simulink model "HANcoder_E407_TTA_Template_DS_V52"  (R2023a)
settings: Solver=FixedStepDiscrete  StartTime=0.0  StopTime=1  FixedStep=0.01  RelTol=1e-3
PreLoadFcn:
  | librarySetup
  | eval([bdroot,'_startup']) %Calling [modelName]_startup.m
values from neighbouring files (symbols this model uses):
  basic_cycle_duration_bc0 = TM_Reset_Board   + COMP_duration    (= 372)    [HANcoder_E407_TTA_Template_DS_V1_startup.m]    (also in HANcoder_E407_TTA_Template_DS_V2_startup.m; HANcoder_E407_TTA_Template_DS_V52_startup.m; HANcoder_E407_TTA_Template_DS_V5_startup.m; HANcoder_E407_TTA_Template_DS_V6_startup.m = 532)
  basic_cycle_duration_bc1 = basic_cycle_duration_bc0    (= 372)    [HANcoder_E407_TTA_Template_DS_V1_startup.m]    (also in HANcoder_E407_TTA_Template_DS_V2_startup.m; HANcoder_E407_TTA_Template_DS_V52_startup.m; HANcoder_E407_TTA_Template_DS_V5_startup.m; HANcoder_E407_TTA_Template_DS_V6_startup.m = 532)
  basic_cycle_duration_bc2 = basic_cycle_duration_bc0    (= 372)    [HANcoder_E407_TTA_Template_DS_V1_startup.m]    (also in HANcoder_E407_TTA_Template_DS_V2_startup.m; HANcoder_E407_TTA_Template_DS_V52_startup.m; HANcoder_E407_TTA_Template_DS_V5_startup.m; HANcoder_E407_TTA_Template_DS_V6_startup.m = 532)
  comm_delay_estimation1 = round(comm_delay_measured1*hardware_granularity/frequency_IRQ)    [HANcoder_E407_TTA_Template_DS_V1_startup.m]    (also in HANcoder_E407_TTA_Template_DS_V2_startup.m; HANcoder_E407_TTA_Template_DS_V52_startup.m; HANcoder_E407_TTA_Template_DS_V5_startup.m; HANcoder_E407_TTA_Template_DS_V6_startup.m)
  comm_delay_estimation2 = round(comm_delay_measured2*hardware_granularity/frequency_IRQ)    [HANcoder_E407_TTA_Template_DS_V1_startup.m]    (also in HANcoder_E407_TTA_Template_DS_V2_startup.m; HANcoder_E407_TTA_Template_DS_V52_startup.m; HANcoder_E407_TTA_Template_DS_V5_startup.m; HANcoder_E407_TTA_Template_DS_V6_startup.m)
  COMM_Period = 80    [HANcoder_E407_TTA_Template_DS_V1_startup.m]    (also in HANcoder_E407_TTA_Template_DS_V2_startup.m; HANcoder_E407_TTA_Template_DS_V52_startup.m; HANcoder_E407_TTA_Template_DS_V5_startup.m; HANcoder_E407_TTA_Template_DS_V6_startup.m = 120)
  COMM_Phase1 = Simulink.Parameter    [HANcoder_E407_TTA_Template_DS_V1_startup.m]    (also in HANcoder_E407_TTA_Template_DS_V2_startup.m; HANcoder_E407_TTA_Template_DS_V52_startup.m; HANcoder_E407_TTA_Template_DS_V5_startup.m; HANcoder_E407_TTA_Template_DS_V6_startup.m)
  COMM_Phase2 = Simulink.Parameter    [HANcoder_E407_TTA_Template_DS_V1_startup.m]    (also in HANcoder_E407_TTA_Template_DS_V2_startup.m; HANcoder_E407_TTA_Template_DS_V52_startup.m; HANcoder_E407_TTA_Template_DS_V5_startup.m; HANcoder_E407_TTA_Template_DS_V6_startup.m)
  COMM_Phase_init1 = Simulink.Parameter    [HANcoder_E407_TTA_Template_DS_V1_startup.m]    (also in HANcoder_E407_TTA_Template_DS_V2_startup.m; HANcoder_E407_TTA_Template_DS_V52_startup.m; HANcoder_E407_TTA_Template_DS_V5_startup.m; HANcoder_E407_TTA_Template_DS_V6_startup.m)
  COMM_Phase_init2 = Simulink.Parameter    [HANcoder_E407_TTA_Template_DS_V1_startup.m]    (also in HANcoder_E407_TTA_Template_DS_V2_startup.m; HANcoder_E407_TTA_Template_DS_V52_startup.m; HANcoder_E407_TTA_Template_DS_V5_startup.m; HANcoder_E407_TTA_Template_DS_V6_startup.m)
  COMP_duration = 4    [HANcoder_E407_TTA_Template_DS_V1_startup.m]    (also in HANcoder_E407_TTA_Template_DS_V2_startup.m; HANcoder_E407_TTA_Template_DS_V52_startup.m; HANcoder_E407_TTA_Template_DS_V5_startup.m; HANcoder_E407_TTA_Template_DS_V6_startup.m)
  frequency_IRQ = 100    [HANcoder_E407_TTA_Template_DS_V1_startup.m]    (also in HANcoder_E407_TTA_Template_DS_V2_startup.m; HANcoder_E407_TTA_Template_DS_V52_startup.m; HANcoder_E407_TTA_Template_DS_V5_startup.m; HANcoder_E407_TTA_Template_DS_V6_startup.m)
  idle_time_init = basic_cycle_duration_bc0 + basic_cycle_duration_bc1    (= 744)    [HANcoder_E407_TTA_Template_DS_V1_startup.m]    (also in HANcoder_E407_TTA_Template_DS_V2_startup.m; HANcoder_E407_TTA_Template_DS_V52_startup.m = 1116; HANcoder_E407_TTA_Template_DS_V5_startup.m = 1116; HANcoder_E407_TTA_Template_DS_V6_startup.m = 1596)
  L0b = 0.5    [HANcoder_E407_TTA_Template_DS_V52_startup.m]    (also in HANcoder_E407_TTA_Template_DS_V5_startup.m; HANcoder_E407_TTA_Template_DS_V6_startup.m)
  L0f = 5    [HANcoder_E407_TTA_Template_DS_V52_startup.m]    (also in HANcoder_E407_TTA_Template_DS_V5_startup.m; HANcoder_E407_TTA_Template_DS_V6_startup.m)
  L1f = 6    [HANcoder_E407_TTA_Template_DS_V52_startup.m]    (also in HANcoder_E407_TTA_Template_DS_V5_startup.m; HANcoder_E407_TTA_Template_DS_V6_startup.m)
  LA_Clock_Gr = 1    [HANcoder_E407_TTA_Template_DS_V1_startup.m]    (also in HANcoder_E407_TTA_Template_DS_V2_startup.m; HANcoder_E407_TTA_Template_DS_V52_startup.m; HANcoder_E407_TTA_Template_DS_V5_startup.m; HANcoder_E407_TTA_Template_DS_V6_startup.m)
  LA_COMM_dly = 1    [HANcoder_E407_TTA_Template_DS_V1_startup.m]    (also in HANcoder_E407_TTA_Template_DS_V2_startup.m; HANcoder_E407_TTA_Template_DS_V52_startup.m; HANcoder_E407_TTA_Template_DS_V5_startup.m; HANcoder_E407_TTA_Template_DS_V6_startup.m)
  LA_COMM_Err = 1    [HANcoder_E407_TTA_Template_DS_V1_startup.m]    (also in HANcoder_E407_TTA_Template_DS_V2_startup.m; HANcoder_E407_TTA_Template_DS_V52_startup.m; HANcoder_E407_TTA_Template_DS_V5_startup.m; HANcoder_E407_TTA_Template_DS_V6_startup.m)
  LA_E_Desync = 1    [HANcoder_E407_TTA_Template_DS_V1_startup.m]    (also in HANcoder_E407_TTA_Template_DS_V2_startup.m; HANcoder_E407_TTA_Template_DS_V52_startup.m; HANcoder_E407_TTA_Template_DS_V5_startup.m; HANcoder_E407_TTA_Template_DS_V6_startup.m)
  LA_MEX_Flag = 1    [HANcoder_E407_TTA_Template_DS_V1_startup.m]    (also in HANcoder_E407_TTA_Template_DS_V2_startup.m; HANcoder_E407_TTA_Template_DS_V52_startup.m; HANcoder_E407_TTA_Template_DS_V5_startup.m; HANcoder_E407_TTA_Template_DS_V6_startup.m)
  LA_Task_Act = 1    [HANcoder_E407_TTA_Template_DS_V1_startup.m]    (also in HANcoder_E407_TTA_Template_DS_V2_startup.m; HANcoder_E407_TTA_Template_DS_V52_startup.m; HANcoder_E407_TTA_Template_DS_V5_startup.m; HANcoder_E407_TTA_Template_DS_V6_startup.m)
  Master_Role = 1    [HANcoder_E407_TTA_Template_DS_V1_startup.m]    (also in HANcoder_E407_TTA_Template_DS_V2_startup.m; HANcoder_E407_TTA_Template_DS_V52_startup.m; HANcoder_E407_TTA_Template_DS_V5_startup.m; HANcoder_E407_TTA_Template_DS_V6_startup.m)
  matrix_rows = 3    [HANcoder_E407_TTA_Template_DS_V1_startup.m]    (also in HANcoder_E407_TTA_Template_DS_V2_startup.m; HANcoder_E407_TTA_Template_DS_V52_startup.m; HANcoder_E407_TTA_Template_DS_V5_startup.m; HANcoder_E407_TTA_Template_DS_V6_startup.m)
  max_desync = 15    [HANcoder_E407_TTA_Template_DS_V1_startup.m]    (also in HANcoder_E407_TTA_Template_DS_V2_startup.m; HANcoder_E407_TTA_Template_DS_V52_startup.m; HANcoder_E407_TTA_Template_DS_V5_startup.m; HANcoder_E407_TTA_Template_DS_V6_startup.m)
  max_num_msgs_CAN1 = 2^Tx_bit_number-1    (= 7)    [HANcoder_E407_TTA_Template_DS_V1_startup.m]    (also in HANcoder_E407_TTA_Template_DS_V2_startup.m; HANcoder_E407_TTA_Template_DS_V52_startup.m; HANcoder_E407_TTA_Template_DS_V5_startup.m; HANcoder_E407_TTA_Template_DS_V6_startup.m)
  max_num_msgs_CAN2 = max_num_msgs_CAN1    (= 7)    [HANcoder_E407_TTA_Template_DS_V1_startup.m]    (also in HANcoder_E407_TTA_Template_DS_V2_startup.m; HANcoder_E407_TTA_Template_DS_V52_startup.m; HANcoder_E407_TTA_Template_DS_V5_startup.m; HANcoder_E407_TTA_Template_DS_V6_startup.m)
  min_desync = (-1)*max_desync    (= -15)    [HANcoder_E407_TTA_Template_DS_V1_startup.m]    (also in HANcoder_E407_TTA_Template_DS_V2_startup.m; HANcoder_E407_TTA_Template_DS_V52_startup.m; HANcoder_E407_TTA_Template_DS_V5_startup.m; HANcoder_E407_TTA_Template_DS_V6_startup.m)
  PID_derivative = Simulink.Parameter    [HANcoder_E407_TTA_Template_DS_V52_startup.m]    (also in HANcoder_E407_TTA_Template_DS_V6_startup.m)
  PID_gain = Simulink.Parameter    [HANcoder_E407_TTA_Template_DS_V52_startup.m]    (also in HANcoder_E407_TTA_Template_DS_V6_startup.m)
  PID_integrator = Simulink.Parameter    [HANcoder_E407_TTA_Template_DS_V52_startup.m]    (also in HANcoder_E407_TTA_Template_DS_V6_startup.m)
  PotValue1_ID = 22    [HANcoder_E407_TTA_Template_DS_V1_startup.m]    (also in HANcoder_E407_TTA_Template_DS_V2_startup.m; HANcoder_E407_TTA_Template_DS_V52_startup.m; HANcoder_E407_TTA_Template_DS_V5_startup.m; HANcoder_E407_TTA_Template_DS_V6_startup.m)
  PotValue2_ID = 23    [HANcoder_E407_TTA_Template_DS_V1_startup.m]    (also in HANcoder_E407_TTA_Template_DS_V2_startup.m; HANcoder_E407_TTA_Template_DS_V52_startup.m; HANcoder_E407_TTA_Template_DS_V5_startup.m; HANcoder_E407_TTA_Template_DS_V6_startup.m)
  PotValue3_ID = 24    [HANcoder_E407_TTA_Template_DS_V1_startup.m]    (also in HANcoder_E407_TTA_Template_DS_V2_startup.m; HANcoder_E407_TTA_Template_DS_V52_startup.m; HANcoder_E407_TTA_Template_DS_V5_startup.m; HANcoder_E407_TTA_Template_DS_V6_startup.m)
  script_run = Simulink.Parameter    [HANcoder_E407_TTA_Template_DS_V1_startup.m]    (also in HANcoder_E407_TTA_Template_DS_V2_startup.m; HANcoder_E407_TTA_Template_DS_V52_startup.m; HANcoder_E407_TTA_Template_DS_V5_startup.m; HANcoder_E407_TTA_Template_DS_V6_startup.m)
  Slave_Role = 2    [HANcoder_E407_TTA_Template_DS_V1_startup.m]    (also in HANcoder_E407_TTA_Template_DS_V2_startup.m; HANcoder_E407_TTA_Template_DS_V52_startup.m; HANcoder_E407_TTA_Template_DS_V5_startup.m; HANcoder_E407_TTA_Template_DS_V6_startup.m)
  Sync_ID = 1    [HANcoder_E407_TTA_Template_DS_V1_startup.m]    (also in HANcoder_E407_TTA_Template_DS_V2_startup.m; HANcoder_E407_TTA_Template_DS_V52_startup.m; HANcoder_E407_TTA_Template_DS_V5_startup.m; HANcoder_E407_TTA_Template_DS_V6_startup.m)
  TM_Check_PotValue1 = TM_COMM_PotValue1 + COMM_duration    (= 174)    [HANcoder_E407_TTA_Template_DS_V1_startup.m]    (also in HANcoder_E407_TTA_Template_DS_V2_startup.m; HANcoder_E407_TTA_Template_DS_V52_startup.m; HANcoder_E407_TTA_Template_DS_V5_startup.m; HANcoder_E407_TTA_Template_DS_V6_startup.m = 254)
  TM_Check_PotValue2 = TM_COMM_PotValue2 + COMM_duration    (= 258)    [HANcoder_E407_TTA_Template_DS_V1_startup.m]    (also in HANcoder_E407_TTA_Template_DS_V2_startup.m; HANcoder_E407_TTA_Template_DS_V52_startup.m; HANcoder_E407_TTA_Template_DS_V5_startup.m; HANcoder_E407_TTA_Template_DS_V6_startup.m = 378)
  TM_Check_PotValue3 = TM_COMM_PotValue3 + COMM_duration    (= 342)    [HANcoder_E407_TTA_Template_DS_V1_startup.m]    (also in HANcoder_E407_TTA_Template_DS_V2_startup.m; HANcoder_E407_TTA_Template_DS_V52_startup.m; HANcoder_E407_TTA_Template_DS_V5_startup.m; HANcoder_E407_TTA_Template_DS_V6_startup.m = 502)
  TM_Check_Sync = TM_COMM_Sync   + COMM_duration    (= 80)    [HANcoder_E407_TTA_Template_DS_V1_startup.m]    (also in HANcoder_E407_TTA_Template_DS_V2_startup.m; HANcoder_E407_TTA_Template_DS_V52_startup.m; HANcoder_E407_TTA_Template_DS_V5_startup.m; HANcoder_E407_TTA_Template_DS_V6_startup.m = 120)
  TM_Check_TOuts = TM_Count_Vote3 + COMP_duration    (= 356)    [HANcoder_E407_TTA_Template_DS_V1_startup.m]    (also in HANcoder_E407_TTA_Template_DS_V2_startup.m; HANcoder_E407_TTA_Template_DS_V52_startup.m; HANcoder_E407_TTA_Template_DS_V5_startup.m; HANcoder_E407_TTA_Template_DS_V6_startup.m = 516)
  TM_Check_Trailer1Articulation = TM_COMM_Trailer1Articulation + COMM_duration    (= 170)    [HANcoder_E407_TTA_Template_DS_V1_startup.m]    (also in HANcoder_E407_TTA_Template_DS_V2_startup.m; HANcoder_E407_TTA_Template_DS_V52_startup.m; HANcoder_E407_TTA_Template_DS_V5_startup.m; HANcoder_E407_TTA_Template_DS_V6_startup.m = 250)
  TM_Check_Trailer2Articulation = TM_COMM_Trailer2Articulation + COMM_duration    (= 254)    [HANcoder_E407_TTA_Template_DS_V1_startup.m]    (also in HANcoder_E407_TTA_Template_DS_V2_startup.m; HANcoder_E407_TTA_Template_DS_V52_startup.m; HANcoder_E407_TTA_Template_DS_V5_startup.m; HANcoder_E407_TTA_Template_DS_V6_startup.m = 374)
  TM_Check_Vote1 = TM_COMM_Vote1  + COMM_duration    (= 172)    [HANcoder_E407_TTA_Template_DS_V1_startup.m]    (also in HANcoder_E407_TTA_Template_DS_V2_startup.m; HANcoder_E407_TTA_Template_DS_V52_startup.m; HANcoder_E407_TTA_Template_DS_V5_startup.m; HANcoder_E407_TTA_Template_DS_V6_startup.m = 252)
  TM_Check_Vote2 = TM_COMM_Vote2  + COMM_duration    (= 260)    [HANcoder_E407_TTA_Template_DS_V1_startup.m]    (also in HANcoder_E407_TTA_Template_DS_V2_startup.m; HANcoder_E407_TTA_Template_DS_V52_startup.m; HANcoder_E407_TTA_Template_DS_V5_startup.m; HANcoder_E407_TTA_Template_DS_V6_startup.m = 380)
  TM_Check_Vote3 = TM_COMM_Vote3  + COMM_duration    (= 348)    [HANcoder_E407_TTA_Template_DS_V1_startup.m]    (also in HANcoder_E407_TTA_Template_DS_V2_startup.m; HANcoder_E407_TTA_Template_DS_V52_startup.m; HANcoder_E407_TTA_Template_DS_V5_startup.m; HANcoder_E407_TTA_Template_DS_V6_startup.m = 508)
  TM_COMM_PotValue1 = TM_ReadPot + COMP_duration    (= 94)    [HANcoder_E407_TTA_Template_DS_V1_startup.m]    (also in HANcoder_E407_TTA_Template_DS_V2_startup.m; HANcoder_E407_TTA_Template_DS_V52_startup.m; HANcoder_E407_TTA_Template_DS_V5_startup.m; HANcoder_E407_TTA_Template_DS_V6_startup.m = 134)
  TM_COMM_PotValue2 = TM_Check_PotValue1 + COMP_duration    (= 178)    [HANcoder_E407_TTA_Template_DS_V1_startup.m]    (also in HANcoder_E407_TTA_Template_DS_V2_startup.m; HANcoder_E407_TTA_Template_DS_V52_startup.m; HANcoder_E407_TTA_Template_DS_V5_startup.m; HANcoder_E407_TTA_Template_DS_V6_startup.m = 258)
  TM_COMM_PotValue3 = TM_Check_PotValue2 + COMP_duration    (= 262)    [HANcoder_E407_TTA_Template_DS_V1_startup.m]    (also in HANcoder_E407_TTA_Template_DS_V2_startup.m; HANcoder_E407_TTA_Template_DS_V52_startup.m; HANcoder_E407_TTA_Template_DS_V5_startup.m; HANcoder_E407_TTA_Template_DS_V6_startup.m = 382)
  TM_COMM_Sync = basic_cycle_start    (= 0)    [HANcoder_E407_TTA_Template_DS_V1_startup.m]    (also in HANcoder_E407_TTA_Template_DS_V2_startup.m; HANcoder_E407_TTA_Template_DS_V52_startup.m; HANcoder_E407_TTA_Template_DS_V5_startup.m; HANcoder_E407_TTA_Template_DS_V6_startup.m)
  TM_COMM_Trailer1Articulation = TM_Update_LT_2 + COMP_duration    (= 90)    [HANcoder_E407_TTA_Template_DS_V1_startup.m]    (also in HANcoder_E407_TTA_Template_DS_V2_startup.m; HANcoder_E407_TTA_Template_DS_V52_startup.m; HANcoder_E407_TTA_Template_DS_V5_startup.m; HANcoder_E407_TTA_Template_DS_V6_startup.m = 130)
  TM_COMM_Trailer2Articulation = TM_Check_Trailer1Articulation + COMP_duration    (= 174)    [HANcoder_E407_TTA_Template_DS_V1_startup.m]    (also in HANcoder_E407_TTA_Template_DS_V2_startup.m; HANcoder_E407_TTA_Template_DS_V52_startup.m; HANcoder_E407_TTA_Template_DS_V5_startup.m; HANcoder_E407_TTA_Template_DS_V6_startup.m = 254)
  TM_COMM_Vote1 = TM_Vote_Dec    + COMP_duration    (= 92)    [HANcoder_E407_TTA_Template_DS_V1_startup.m]    (also in HANcoder_E407_TTA_Template_DS_V2_startup.m; HANcoder_E407_TTA_Template_DS_V52_startup.m; HANcoder_E407_TTA_Template_DS_V5_startup.m; HANcoder_E407_TTA_Template_DS_V6_startup.m = 132)
  TM_COMM_Vote2 = TM_Count_Vote1 + COMP_duration    (= 180)    [HANcoder_E407_TTA_Template_DS_V1_startup.m]    (also in HANcoder_E407_TTA_Template_DS_V2_startup.m; HANcoder_E407_TTA_Template_DS_V52_startup.m; HANcoder_E407_TTA_Template_DS_V5_startup.m; HANcoder_E407_TTA_Template_DS_V6_startup.m = 260)
  TM_COMM_Vote3 = TM_Count_Vote2 + COMP_duration    (= 268)    [HANcoder_E407_TTA_Template_DS_V1_startup.m]    (also in HANcoder_E407_TTA_Template_DS_V2_startup.m; HANcoder_E407_TTA_Template_DS_V52_startup.m; HANcoder_E407_TTA_Template_DS_V5_startup.m; HANcoder_E407_TTA_Template_DS_V6_startup.m = 388)
  TM_Count_Vote1 = TM_Check_Vote1 + COMP_duration    (= 176)    [HANcoder_E407_TTA_Template_DS_V1_startup.m]    (also in HANcoder_E407_TTA_Template_DS_V2_startup.m; HANcoder_E407_TTA_Template_DS_V52_startup.m; HANcoder_E407_TTA_Template_DS_V5_startup.m; HANcoder_E407_TTA_Template_DS_V6_startup.m = 256)
  TM_Count_Vote2 = TM_Check_Vote2 + COMP_duration    (= 264)    [HANcoder_E407_TTA_Template_DS_V1_startup.m]    (also in HANcoder_E407_TTA_Template_DS_V2_startup.m; HANcoder_E407_TTA_Template_DS_V52_startup.m; HANcoder_E407_TTA_Template_DS_V5_startup.m; HANcoder_E407_TTA_Template_DS_V6_startup.m = 384)
  TM_Count_Vote3 = TM_Check_Vote3 + COMP_duration    (= 352)    [HANcoder_E407_TTA_Template_DS_V1_startup.m]    (also in HANcoder_E407_TTA_Template_DS_V2_startup.m; HANcoder_E407_TTA_Template_DS_V52_startup.m; HANcoder_E407_TTA_Template_DS_V5_startup.m; HANcoder_E407_TTA_Template_DS_V6_startup.m = 512)
  TM_Data_bc0 = TM_COMM_Sync    (= 0)    [HANcoder_E407_TTA_Template_DS_V1_startup.m]    (also in HANcoder_E407_TTA_Template_DS_V2_startup.m; HANcoder_E407_TTA_Template_DS_V52_startup.m; HANcoder_E407_TTA_Template_DS_V5_startup.m; HANcoder_E407_TTA_Template_DS_V6_startup.m)
  TM_Data_bc1 = TM_Data_bc0(1:4)    [HANcoder_E407_TTA_Template_DS_V1_startup.m]    (also in HANcoder_E407_TTA_Template_DS_V2_startup.m; HANcoder_E407_TTA_Template_DS_V52_startup.m; HANcoder_E407_TTA_Template_DS_V5_startup.m; HANcoder_E407_TTA_Template_DS_V6_startup.m)
  TM_Data_bc2 = TM_Data_bc0(1:4)    [HANcoder_E407_TTA_Template_DS_V1_startup.m]    (also in HANcoder_E407_TTA_Template_DS_V2_startup.m; HANcoder_E407_TTA_Template_DS_V52_startup.m; HANcoder_E407_TTA_Template_DS_V5_startup.m; HANcoder_E407_TTA_Template_DS_V6_startup.m)
  TM_InverseKinematics = TM_Check_Trailer2Articulation + COMP_duration    (= 258)    [HANcoder_E407_TTA_Template_DS_V1_startup.m]    (also in HANcoder_E407_TTA_Template_DS_V2_startup.m; HANcoder_E407_TTA_Template_DS_V52_startup.m; HANcoder_E407_TTA_Template_DS_V5_startup.m; HANcoder_E407_TTA_Template_DS_V6_startup.m = 378)
  TM_New_Master = TM_Check_TOuts + COMP_duration    (= 360)    [HANcoder_E407_TTA_Template_DS_V1_startup.m]    (also in HANcoder_E407_TTA_Template_DS_V2_startup.m; HANcoder_E407_TTA_Template_DS_V52_startup.m; HANcoder_E407_TTA_Template_DS_V5_startup.m; HANcoder_E407_TTA_Template_DS_V6_startup.m = 520)
  TM_PotVote = TM_COMM_PotValue3 + COMP_duration    (= 266)    [HANcoder_E407_TTA_Template_DS_V1_startup.m]    (also in HANcoder_E407_TTA_Template_DS_V2_startup.m; HANcoder_E407_TTA_Template_DS_V52_startup.m; HANcoder_E407_TTA_Template_DS_V5_startup.m; HANcoder_E407_TTA_Template_DS_V6_startup.m = 386)
  TM_ReadPot = TM_Update_LT_2 + COMP_duration    (= 90)    [HANcoder_E407_TTA_Template_DS_V1_startup.m]    (also in HANcoder_E407_TTA_Template_DS_V2_startup.m; HANcoder_E407_TTA_Template_DS_V52_startup.m; HANcoder_E407_TTA_Template_DS_V5_startup.m; HANcoder_E407_TTA_Template_DS_V6_startup.m = 130)
  TM_Reset_Board = TM_Reset_Var   + COMP_duration    (= 368)    [HANcoder_E407_TTA_Template_DS_V1_startup.m]    (also in HANcoder_E407_TTA_Template_DS_V2_startup.m; HANcoder_E407_TTA_Template_DS_V52_startup.m; HANcoder_E407_TTA_Template_DS_V5_startup.m; HANcoder_E407_TTA_Template_DS_V6_startup.m = 528)
  TM_Reset_Var = TM_New_Master  + COMP_duration    (= 364)    [HANcoder_E407_TTA_Template_DS_V1_startup.m]    (also in HANcoder_E407_TTA_Template_DS_V2_startup.m; HANcoder_E407_TTA_Template_DS_V52_startup.m; HANcoder_E407_TTA_Template_DS_V5_startup.m; HANcoder_E407_TTA_Template_DS_V6_startup.m = 524)
  TM_Reset_Var_bc1 = TM_Data_bc1(end) + COMP_duration    [HANcoder_E407_TTA_Template_DS_V1_startup.m]    (also in HANcoder_E407_TTA_Template_DS_V2_startup.m; HANcoder_E407_TTA_Template_DS_V52_startup.m; HANcoder_E407_TTA_Template_DS_V5_startup.m; HANcoder_E407_TTA_Template_DS_V6_startup.m)
  TM_Reset_Var_bc1_2 = TM_Reset_Var_bc1 +2    [HANcoder_E407_TTA_Template_DS_V1_startup.m]    (also in HANcoder_E407_TTA_Template_DS_V2_startup.m; HANcoder_E407_TTA_Template_DS_V52_startup.m; HANcoder_E407_TTA_Template_DS_V5_startup.m; HANcoder_E407_TTA_Template_DS_V6_startup.m)
  TM_Reset_Var_bc2 = TM_Data_bc2(end) + COMP_duration    [HANcoder_E407_TTA_Template_DS_V1_startup.m]    (also in HANcoder_E407_TTA_Template_DS_V2_startup.m; HANcoder_E407_TTA_Template_DS_V52_startup.m; HANcoder_E407_TTA_Template_DS_V5_startup.m; HANcoder_E407_TTA_Template_DS_V6_startup.m)
  TM_Reset_Var_bc2_2 = TM_Reset_Var_bc2 +2    [HANcoder_E407_TTA_Template_DS_V1_startup.m]    (also in HANcoder_E407_TTA_Template_DS_V2_startup.m; HANcoder_E407_TTA_Template_DS_V52_startup.m; HANcoder_E407_TTA_Template_DS_V5_startup.m; HANcoder_E407_TTA_Template_DS_V6_startup.m)
  TM_SteerControl = TM_InverseKinematics + COMP_duration    (= 262)    [HANcoder_E407_TTA_Template_DS_V1_startup.m]    (also in HANcoder_E407_TTA_Template_DS_V2_startup.m; HANcoder_E407_TTA_Template_DS_V52_startup.m = 259; HANcoder_E407_TTA_Template_DS_V5_startup.m = 259)
  TM_Type_bc0 = COMM    (= 0)    [HANcoder_E407_TTA_Template_DS_V1_startup.m]    (also in HANcoder_E407_TTA_Template_DS_V2_startup.m; HANcoder_E407_TTA_Template_DS_V52_startup.m; HANcoder_E407_TTA_Template_DS_V5_startup.m; HANcoder_E407_TTA_Template_DS_V6_startup.m)
  TM_Type_bc1 = TM_Type_bc0(1:4)    [HANcoder_E407_TTA_Template_DS_V1_startup.m]    (also in HANcoder_E407_TTA_Template_DS_V2_startup.m; HANcoder_E407_TTA_Template_DS_V52_startup.m; HANcoder_E407_TTA_Template_DS_V5_startup.m; HANcoder_E407_TTA_Template_DS_V6_startup.m)
  TM_Type_bc2 = TM_Type_bc0(1:4)    [HANcoder_E407_TTA_Template_DS_V1_startup.m]    (also in HANcoder_E407_TTA_Template_DS_V2_startup.m; HANcoder_E407_TTA_Template_DS_V52_startup.m; HANcoder_E407_TTA_Template_DS_V5_startup.m; HANcoder_E407_TTA_Template_DS_V6_startup.m)
  TM_Update_LT = TM_Check_Sync  + COMP_duration    (= 84)    [HANcoder_E407_TTA_Template_DS_V1_startup.m]    (also in HANcoder_E407_TTA_Template_DS_V2_startup.m; HANcoder_E407_TTA_Template_DS_V52_startup.m; HANcoder_E407_TTA_Template_DS_V5_startup.m; HANcoder_E407_TTA_Template_DS_V6_startup.m = 124)
  TM_Update_LT_2 = TM_Update_LT   + 2    (= 86)    [HANcoder_E407_TTA_Template_DS_V1_startup.m]    (also in HANcoder_E407_TTA_Template_DS_V2_startup.m; HANcoder_E407_TTA_Template_DS_V52_startup.m; HANcoder_E407_TTA_Template_DS_V5_startup.m; HANcoder_E407_TTA_Template_DS_V6_startup.m = 126)
  TM_Vote_Dec = TM_Update_LT   + COMP_duration    (= 88)    [HANcoder_E407_TTA_Template_DS_V1_startup.m]    (also in HANcoder_E407_TTA_Template_DS_V2_startup.m; HANcoder_E407_TTA_Template_DS_V52_startup.m; HANcoder_E407_TTA_Template_DS_V5_startup.m; HANcoder_E407_TTA_Template_DS_V6_startup.m = 128)
  Tractor_Board1 = 11    [HANcoder_E407_TTA_Template_DS_V1_startup.m]    (also in HANcoder_E407_TTA_Template_DS_V2_startup.m = 1; HANcoder_E407_TTA_Template_DS_V52_startup.m = 1; HANcoder_E407_TTA_Template_DS_V5_startup.m = 1; HANcoder_E407_TTA_Template_DS_V6_startup.m = 1)
  Tractor_Board2 = 12    [HANcoder_E407_TTA_Template_DS_V1_startup.m]    (also in HANcoder_E407_TTA_Template_DS_V2_startup.m = 2; HANcoder_E407_TTA_Template_DS_V52_startup.m = 2; HANcoder_E407_TTA_Template_DS_V5_startup.m = 2; HANcoder_E407_TTA_Template_DS_V6_startup.m = 2)
  Tractor_Board3 = 13    [HANcoder_E407_TTA_Template_DS_V1_startup.m]    (also in HANcoder_E407_TTA_Template_DS_V2_startup.m = 3; HANcoder_E407_TTA_Template_DS_V52_startup.m = 3; HANcoder_E407_TTA_Template_DS_V5_startup.m = 3; HANcoder_E407_TTA_Template_DS_V6_startup.m = 3)
  Trailer1_Articulation_ID = 31    [HANcoder_E407_TTA_Template_DS_V1_startup.m]    (also in HANcoder_E407_TTA_Template_DS_V2_startup.m; HANcoder_E407_TTA_Template_DS_V52_startup.m; HANcoder_E407_TTA_Template_DS_V5_startup.m; HANcoder_E407_TTA_Template_DS_V6_startup.m)
  Trailer1_Board1 = 2    [HANcoder_E407_TTA_Template_DS_V1_startup.m]    (also in HANcoder_E407_TTA_Template_DS_V2_startup.m = 4; HANcoder_E407_TTA_Template_DS_V52_startup.m = 4; HANcoder_E407_TTA_Template_DS_V5_startup.m = 4; HANcoder_E407_TTA_Template_DS_V6_startup.m = 4)
  Trailer1_Board2 = 3    [HANcoder_E407_TTA_Template_DS_V1_startup.m]    (also in HANcoder_E407_TTA_Template_DS_V2_startup.m = 5; HANcoder_E407_TTA_Template_DS_V52_startup.m = 5; HANcoder_E407_TTA_Template_DS_V5_startup.m = 5; HANcoder_E407_TTA_Template_DS_V6_startup.m = 5)
  Trailer1_Board3 = 4    [HANcoder_E407_TTA_Template_DS_V1_startup.m]    (also in HANcoder_E407_TTA_Template_DS_V2_startup.m = 6; HANcoder_E407_TTA_Template_DS_V52_startup.m = 6; HANcoder_E407_TTA_Template_DS_V5_startup.m = 6; HANcoder_E407_TTA_Template_DS_V6_startup.m = 6)
  Trailer2_Articulation_ID = 32    [HANcoder_E407_TTA_Template_DS_V1_startup.m]    (also in HANcoder_E407_TTA_Template_DS_V2_startup.m; HANcoder_E407_TTA_Template_DS_V52_startup.m; HANcoder_E407_TTA_Template_DS_V5_startup.m; HANcoder_E407_TTA_Template_DS_V6_startup.m)
  Trailer2_Board1 = 5    [HANcoder_E407_TTA_Template_DS_V1_startup.m]    (also in HANcoder_E407_TTA_Template_DS_V2_startup.m = 7; HANcoder_E407_TTA_Template_DS_V52_startup.m = 7; HANcoder_E407_TTA_Template_DS_V5_startup.m = 7; HANcoder_E407_TTA_Template_DS_V6_startup.m = 7)
  Trailer2_Board2 = 6    [HANcoder_E407_TTA_Template_DS_V1_startup.m]    (also in HANcoder_E407_TTA_Template_DS_V2_startup.m = 8; HANcoder_E407_TTA_Template_DS_V52_startup.m = 8; HANcoder_E407_TTA_Template_DS_V5_startup.m = 8; HANcoder_E407_TTA_Template_DS_V6_startup.m = 8)
  Trailer2_Board3 = 7    [HANcoder_E407_TTA_Template_DS_V1_startup.m]    (also in HANcoder_E407_TTA_Template_DS_V2_startup.m = 9; HANcoder_E407_TTA_Template_DS_V52_startup.m = 9; HANcoder_E407_TTA_Template_DS_V5_startup.m = 9; HANcoder_E407_TTA_Template_DS_V6_startup.m = 9)
  V1 = -0.000000001    (= -1e-09)    [HANcoder_E407_TTA_Template_DS_V52_startup.m]    (also in HANcoder_E407_TTA_Template_DS_V5_startup.m; HANcoder_E407_TTA_Template_DS_V6_startup.m)
  V2 = -0.000000001    (= -1e-09)    [HANcoder_E407_TTA_Template_DS_V52_startup.m]    (also in HANcoder_E407_TTA_Template_DS_V5_startup.m; HANcoder_E407_TTA_Template_DS_V6_startup.m)
  Vote1_ID = 11    [HANcoder_E407_TTA_Template_DS_V1_startup.m]    (also in HANcoder_E407_TTA_Template_DS_V2_startup.m; HANcoder_E407_TTA_Template_DS_V52_startup.m; HANcoder_E407_TTA_Template_DS_V5_startup.m; HANcoder_E407_TTA_Template_DS_V6_startup.m)
  Vote2_ID = 12    [HANcoder_E407_TTA_Template_DS_V1_startup.m]    (also in HANcoder_E407_TTA_Template_DS_V2_startup.m; HANcoder_E407_TTA_Template_DS_V52_startup.m; HANcoder_E407_TTA_Template_DS_V5_startup.m; HANcoder_E407_TTA_Template_DS_V6_startup.m)
  Vote3_ID = 13    [HANcoder_E407_TTA_Template_DS_V1_startup.m]    (also in HANcoder_E407_TTA_Template_DS_V2_startup.m; HANcoder_E407_TTA_Template_DS_V52_startup.m; HANcoder_E407_TTA_Template_DS_V5_startup.m; HANcoder_E407_TTA_Template_DS_V6_startup.m)
undefined symbols (not defined in the file or in its folder): A0, A1, A2, A3, A4, A5, CON2, CON3, CON4, D10, D12, D13, D6, D7, D8, D9
libraries: hdlsllib x136, simulink x39, HANcoder_STM32_Target x31, simulink_extras x8, dspstat3 x2, slpidlib x1
(part 33 of 40)

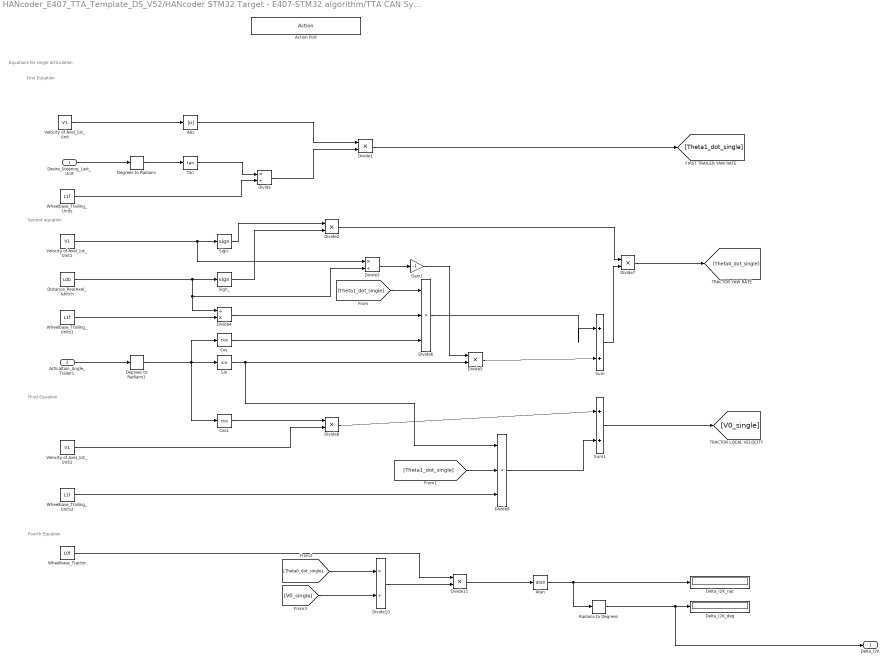
== system HANcoder_E407_TTA_Template_DS_V52/HANcoder STM32 Target - E407-STM32 algorithm/TTA CAN System/TTA System/Matrix Cycle Manager/Controller Matrix Cycle/controller basic cycle 2/COMP Task - Inverse Kinematics Model/Enabled Subsystem/Single Articulation Subsystem ==
  note: Equations for single Articulation
  note: Third Equation
  note: Fourth Equation
  note: Second equation
  note: First Equation
  Desire_Steering_Last_Unit : Inport
  Articaltion_Angle_Trailer1 : Inport  Port=2
  Action Port : ActionPort  ActionPortLabel=case [ 1 ]:
  Abs : Abs  SaturateOnIntegerOverflow=off
  Atan : Trigonometry  Operator=atan
  Cos : Trigonometry  Operator=cos
  Cos1 : Trigonometry  Operator=cos
  Degrees to Radians : simulink_extras/Transformations/Degrees to Radians
  Degrees to Radians1 : simulink_extras/Transformations/Degrees to Radians
  Delta_I2K_deg : Display
  Delta_I2K_rad : Display
  Distance_RearAxel_&hitch : Constant  Value=L0b
  Divide : Product  Inputs=*/
  Divide{1..2,5,7..8,11} (6 alike) : Product  Inputs=**
  Divide10 : Product  Inputs=*/
  Divide3 : Product  Inputs=*/
  Divide4 : Product  Inputs=/*
  Divide6 : Product  Inputs=***
  Divide9 : Product  Inputs=***
  Gain1 : Gain  Gain=-1
  Radians to Degrees : simulink_extras/Transformations/Radians to Degrees
  Sign- : Signum
  Sign_ : Signum
  Sin : Trigonometry
  Sum : Sum  Inputs=|++
  Sum1 : Sum  Inputs=|++
  Tan : Trigonometry  Operator=tan
  Velocity of Axel_1st_Unit : Constant  Value=V1
  Velocity of Axel_1st_Unit1 : Constant  Value=V1
  Velocity of Axel_1st_Unit2 : Constant  Value=V1
  Wheelbase_Tractor : Constant  Value=L0f
  Wheelbase_Trailing_Units : Constant  Value=L1f
  Wheelbase_Trailing_Units1 : Constant  Value=L1f
  Wheelbase_Trailing_Units2 : Constant  Value=L1f
  Delta_I2K : Outport
  wires:
  Divide8/1 -> Sum1/1
  [Theta1_dot_single] -> Divide6/1
  Cos1/1 -> Divide8/1
  Divide11/1 -> Atan/1
  Sum/1 -> Divide7/2
  Velocity of Axel_1st_Unit/1 -> Abs/1
  Wheelbase_Trailing_Units1/1 -> Divide4/2
  [V0_single] -> Divide10/2
  Divide5/1 -> Sum/2
  Divide3/1 -> Gain1/1
  Sum1/1 -> [V0_single]
  Divide9/1 -> Sum1/2
  Divide7/1 -> [Theta0_dot_single]
  Divide2/1 -> Divide7/1
  Gain1/1 -> Divide5/1
  [Theta0_dot_single] -> Divide10/1
  Abs/1 -> Divide1/1
  Divide4/1 -> Divide6/2
  Sign_/1 -> Divide2/2
  Wheelbase_Trailing_Units2/1 -> Divide9/3
  Velocity of Axel_1st_Unit2/1 -> Divide8/2
  Divide6/1 -> Sum/1
  Articaltion_Angle_Trailer1/1 -> Degrees to Radians1/1
  Atan/1 -> Radians to Degrees/1, Delta_I2K_rad/1
  Cos/1 -> Divide6/3
  Sin/1 -> Divide9/1, Divide5/2
  Divide10/1 -> Divide11/2
  Sign-/1 -> Divide2/1
  Distance_RearAxel_&hitch/1 -> Divide4/1, Divide3/2, Sign_/1
  Wheelbase_Trailing_Units/1 -> Divide/2
  [Theta1_dot_single] -> Divide9/2
  Wheelbase_Tractor/1 -> Divide11/1
  Divide/1 -> Divide1/2
  Desire_Steering_Last_Unit/1 -> Degrees to Radians/1
  Tan/1 -> Divide/1
  Velocity of Axel_1st_Unit1/1 -> Divide3/1, Sign-/1
  Divide1/1 -> [Theta1_dot_single]
  Radians to Degrees/1 -> Delta_I2K/1, Delta_I2K_deg/1
  Degrees to Radians/1 -> Tan/1
  Degrees to Radians1/1 -> Sin/1, Cos1/1, Cos/1

== system HANcoder_E407_TTA_Template_DS_V52/HANcoder STM32 Target - E407-STM32 algorithm/TTA CAN System/TTA System/Matrix Cycle Manager/Controller Matrix Cycle/controller basic cycle 2/COMP Task - Rx_PotValues2_check/Process_Messages/Demux message CAN1 and check coherence ==
  CAN1_Rx_msg : Inport  OutDataTypeStr=Bus: msg_buffer_type
  expected_basic_cycle : Inport  Port=2
  Enable : EnablePort
  Bus Creator : BusCreator  Inputs=8  OutDataTypeStr=Bus: msg_buffer_type
  Bus Selector : BusSelector  OutputSignals=Buffer_1,Buffer_2,Buffer_3,Buffer_4,Buffer_5,Buffer_6,Buffer_7,Buffer_8
  Constant : Constant  Value=0  OutDataTypeStr=uint8
  Equal1 : RelationalOperator  Operator===  OutDataTypeStr=boolean  RndMeth=Simplest  InputSameDT=off
  Subsystem : Subsystem
  Terminator : Terminator
  msg_count>2_DEBUG : Subsystem
  CAN1_msg : Outport  OutDataTypeStr=Bus: msg_buffer_type  VectorParamsAs1DForOutWhenUnconnected=off
  Msg_Count_CAN1 : Outport  Port=2  VectorParamsAs1DForOutWhenUnconnected=off
  CAN1_msg_coherent : Outport  Port=3  OutputWhenDisabled=reset  InitialOutput=0  VectorParamsAs1DForOutWhenUnconnected=off
  wires:
  Bus Selector/2 -> Bus Creator/2  "<Buffer_2>"
  Bus Selector/3 -> Bus Creator/3  "<Buffer_3>"
  CAN1_Rx_msg/1 -> Bus Selector/1
  Equal1/1 -> CAN1_msg_coherent/1
  expected_basic_cycle/1 -> Equal1/2
  Bus Selector/6 -> Bus Creator/6  "<Buffer_6>"
  Bus Selector/5 -> Bus Creator/5  "<Buffer_5>"
  Bus Selector/7 -> Bus Creator/7  "<Buffer_7>"
  Bus Selector/8 -> Bus Creator/8  "<Buffer_8>"
  Bus Selector/4 -> Bus Creator/4  "<Buffer_4>"
  Bus Selector/1 -> Subsystem/1(Msg_Temporal_Data)  "<Buffer_1>"
  Subsystem/1(basic_cycle) -> Equal1/1
  Subsystem/2(msg_count) -> msg_count>2_DEBUG/1(msg_c), Msg_Count_CAN1/1
  Bus Creator/1 -> CAN1_msg/1
  Constant/1 -> Bus Creator/1
  Subsystem/3(board_id) -> Terminator/1

== system HANcoder_E407_TTA_Template_DS_V52/HANcoder STM32 Target - E407-STM32 algorithm/TTA CAN System/TTA System/Matrix Cycle Manager/Controller Matrix Cycle/controller basic cycle 2/COMP Task - Rx_PotValues2_check/Process_Messages/Demux message CAN1 and check coherence1 ==
  CAN2_Rx_msg : Inport  OutDataTypeStr=Bus: msg_buffer_type
  expected_basic_cycle : Inport  Port=2
  Enable : EnablePort
  Bus Creator : BusCreator  Inputs=8  OutDataTypeStr=Bus: msg_buffer_type
  Bus Selector : BusSelector  OutputSignals=Buffer_1,Buffer_2,Buffer_3,Buffer_4,Buffer_5,Buffer_6,Buffer_7,Buffer_8
  Constant : Constant  Value=0  OutDataTypeStr=uint8
  Equal1 : RelationalOperator  Operator===  OutDataTypeStr=boolean  RndMeth=Simplest  InputSameDT=off
  Subsystem : Subsystem
  Terminator : Terminator
  msg_count>2_DEBUG : Subsystem
  CAN2_msg_coherent : Outport  OutputWhenDisabled=reset  InitialOutput=0  VectorParamsAs1DForOutWhenUnconnected=off
  Msg_Count_CAN2 : Outport  Port=2  VectorParamsAs1DForOutWhenUnconnected=off
  CAN2_msg : Outport  Port=3  OutDataTypeStr=Bus: msg_buffer_type  VectorParamsAs1DForOutWhenUnconnected=off
  wires:
  Bus Selector/2 -> Bus Creator/2  "<Buffer_2>"
  Bus Selector/3 -> Bus Creator/3  "<Buffer_3>"
  CAN2_Rx_msg/1 -> Bus Selector/1
  Equal1/1 -> CAN2_msg_coherent/1
  expected_basic_cycle/1 -> Equal1/2
  Bus Selector/6 -> Bus Creator/6  "<Buffer_6>"
  Bus Selector/5 -> Bus Creator/5  "<Buffer_5>"
  Bus Selector/7 -> Bus Creator/7  "<Buffer_7>"
  Bus Selector/8 -> Bus Creator/8  "<Buffer_8>"
  Bus Selector/4 -> Bus Creator/4  "<Buffer_4>"
  Bus Selector/1 -> Subsystem/1(Msg_Temporal_Data)  "<Buffer_1>"
  Subsystem/1(basic_cycle) -> Equal1/1
  Subsystem/2(msg_count) -> Msg_Count_CAN2/1, msg_count>2_DEBUG/1(msg_c)
  Bus Creator/1 -> CAN2_msg/1
  Constant/1 -> Bus Creator/1
  Subsystem/3(board_id) -> Terminator/1

== system HANcoder_E407_TTA_Template_DS_V52/HANcoder STM32 Target - E407-STM32 algorithm/TTA CAN System/TTA System/Matrix Cycle Manager/Controller Matrix Cycle/controller basic cycle 2/COMP Task - Rx_PotValues2_check/Process_Messages/Desync calculation ==
  note: Estimation of the Local Time when the message was sent
  note: Desync CAN2
      | expected RX - Actual RX
  note: Desync CAN1
      | expected RX - Actual RX
  TM_COMM : Inport
  New_msg_CAN1 : Inport  Port=2
  msg_count_CAN1 : Inport  Port=3
  msg_count_CAN2 : Inport  Port=4
  Enable : EnablePort
  Constant : Constant  Value=COMM_Phase1
  Constant1 : Constant  Value=COMM_Phase2
  Data Store Read : DataStoreRead  DataStoreName=Msg_Rx_Ticks_CAN1  IndexOptions=Index vector (dialog)  Indices=1  OutputSizes=1
  Data Store Read1 : DataStoreRead  DataStoreName=Msg_Rx_Ticks_CAN2  IndexOptions=Index vector (dialog)  Indices=1  OutputSizes=1
  Data Store Write1 : DataStoreWrite  Priority=23  DataStoreName=Desync_Ticks  IndexOptions=Index vector (dialog)  Indices=1  OutputSizes=1
  Minus : Sum  Priority=21  Inputs=+-
  Minus1 : Sum  Priority=20  Inputs=+-
  Multiply : Product  Priority=10
  Multiply1 : Product  Priority=12
  Saturation : Saturate  UpperLimit=max_desync  LowerLimit=min_desync
  Sum : Sum  Priority=11  Inputs=+++
  Sum1 : Sum  Priority=13  Inputs=+++
  Switch1 : Switch  Priority=22  Criteria=u2 > Threshold  SaturateOnIntegerOverflow=off  InputSameDT=off
  delay_estimation_1 : Constant  Value=comm_delay_estimation1
  delay_estimation_2 : Constant  Value=comm_delay_estimation2
  wires:
  TM_COMM/1 -> Sum1/2, Sum/2
  delay_estimation_1/1 -> Sum/3
  msg_count_CAN1/1 -> Multiply/2
  Switch1/1 -> Saturation/1
  Minus/1 -> Switch1/3
  Sum1/1 -> [expected_LT_CAN2]
  delay_estimation_2/1 -> Sum1/3
  Multiply1/1 -> Sum1/1
  [expected_LT_CAN1] -> Minus1/1
  [expected_LT_CAN2] -> Minus/1
  Data Store Read1/1 -> Minus/2
  Multiply/1 -> Sum/1
  Data Store Read/1 -> Minus1/2
  msg_count_CAN2/1 -> Multiply1/2
  Sum/1 -> [expected_LT_CAN1]
  Minus1/1 -> Switch1/1
  Constant/1 -> Multiply/1
  Constant1/1 -> Multiply1/1
  New_msg_CAN1/1 -> Switch1/2
  Saturation/1 -> Data Store Write1/1

== system HANcoder_E407_TTA_Template_DS_V52/HANcoder STM32 Target - E407-STM32 algorithm/TTA CAN System/TTA System/Matrix Cycle Manager/Controller Matrix Cycle/controller basic cycle 2/COMP Task - Rx_PotValues2_check/Process_Messages/Member Counter ==
  Enable : EnablePort
  AND : Logic  IconShape=distinctive  AllPortsSameDT=off  OutDataTypeStr=boolean
  AND1 : Logic  IconShape=distinctive  AllPortsSameDT=off  OutDataTypeStr=boolean
  Add : Sum
  Assign Trailer 2 as Member 1 : Subsystem
  Assign Trailer 2 as Member 2 : Subsystem
  Constant{,1,3..4} (4 alike) : Constant
  Constant2 : Constant  Value=2
  Data Store Read : DataStoreRead  DataStoreName=Members_Nr  IndexOptions=Index vector (dialog)  Indices=1  OutputSizes=1
  Data Store Read1 : DataStoreRead  DataStoreName=Prev_Member1  IndexOptions=Index vector (dialog)  Indices=1  OutputSizes=1
  Data Store Read2 : DataStoreRead  DataStoreName=Prev_Member2  IndexOptions=Index vector (dialog)  Indices=1  OutputSizes=1
  Data Store Write : DataStoreWrite  DataStoreName=Members_Nr  IndexOptions=Index vector (dialog)  Indices=1  OutputSizes=1
  Data Store Write1 : DataStoreWrite  DataStoreName=Member_Counter_Flag  IndexOptions=Index vector (dialog)  Indices=1  OutputSizes=1
  Equal : RelationalOperator  Operator===  OutDataTypeStr=boolean  RndMeth=Simplest  InputSameDT=off
  Equal1 : RelationalOperator  Operator===  OutDataTypeStr=boolean  RndMeth=Simplest  InputSameDT=off
  NotEqual : RelationalOperator  Operator=~=  OutDataTypeStr=boolean  RndMeth=Simplest  InputSameDT=off
  NotEqual1 : RelationalOperator  Operator=~=  OutDataTypeStr=boolean  RndMeth=Simplest  InputSameDT=off
  wires:
  Data Store Read/1 -> Add/1
  Constant/1 -> Data Store Write1/1, Add/2
  Add/1 -> Equal1/1, Equal/1, Data Store Write/1
  Constant1/1 -> Equal/2
  Constant2/1 -> Equal1/2
  Data Store Read1/1 -> NotEqual/1
  Constant3/1 -> NotEqual/2
  AND/1 -> Assign Trailer 2 as Member 1/Enable
  NotEqual/1 -> AND/1
  Equal/1 -> AND/2
  AND1/1 -> Assign Trailer 2 as Member 2/Enable
  Data Store Read2/1 -> NotEqual1/1
  Constant4/1 -> NotEqual1/2
  NotEqual1/1 -> AND1/1
  Equal1/1 -> AND1/2

== system HANcoder_E407_TTA_Template_DS_V52/HANcoder STM32 Target - E407-STM32 algorithm/TTA CAN System/TTA System/Matrix Cycle Manager/Controller Matrix Cycle/controller basic cycle 2/COMP Task - Rx_Trailer1Articulation_check/Process_Messages/Demux message CAN1 and check coherence ==
  CAN1_Rx_msg : Inport  OutDataTypeStr=Bus: msg_buffer_type
  expected_basic_cycle : Inport  Port=2
  Enable : EnablePort
  Bus Creator : BusCreator  Inputs=8  OutDataTypeStr=Bus: msg_buffer_type
  Bus Selector : BusSelector  OutputSignals=Buffer_1,Buffer_2,Buffer_3,Buffer_4,Buffer_5,Buffer_6,Buffer_7,Buffer_8
  Constant : Constant  Value=0  OutDataTypeStr=uint8
  Equal1 : RelationalOperator  Operator===  OutDataTypeStr=boolean  RndMeth=Simplest  InputSameDT=off
  Subsystem : Subsystem
  Terminator : Terminator
  msg_count>2_DEBUG : Subsystem
  CAN1_msg : Outport  OutDataTypeStr=Bus: msg_buffer_type  VectorParamsAs1DForOutWhenUnconnected=off
  Msg_Count_CAN1 : Outport  Port=2  VectorParamsAs1DForOutWhenUnconnected=off
  CAN1_msg_coherent : Outport  Port=3  OutputWhenDisabled=reset  InitialOutput=0  VectorParamsAs1DForOutWhenUnconnected=off
  wires:
  Bus Selector/2 -> Bus Creator/2  "<Buffer_2>"
  Bus Selector/3 -> Bus Creator/3  "<Buffer_3>"
  CAN1_Rx_msg/1 -> Bus Selector/1
  Equal1/1 -> CAN1_msg_coherent/1
  expected_basic_cycle/1 -> Equal1/2
  Bus Selector/6 -> Bus Creator/6  "<Buffer_6>"
  Bus Selector/5 -> Bus Creator/5  "<Buffer_5>"
  Bus Selector/7 -> Bus Creator/7  "<Buffer_7>"
  Bus Selector/8 -> Bus Creator/8  "<Buffer_8>"
  Bus Selector/4 -> Bus Creator/4  "<Buffer_4>"
  Bus Selector/1 -> Subsystem/1(Msg_Temporal_Data)  "<Buffer_1>"
  Subsystem/1(basic_cycle) -> Equal1/1  "basic_cycle_RX_Art1_CAN1"
  Subsystem/2(msg_count) -> msg_count>2_DEBUG/1(msg_c), Msg_Count_CAN1/1
  Bus Creator/1 -> CAN1_msg/1
  Constant/1 -> Bus Creator/1
  Subsystem/3(board_id) -> Terminator/1

== system HANcoder_E407_TTA_Template_DS_V52/HANcoder STM32 Target - E407-STM32 algorithm/TTA CAN System/TTA System/Matrix Cycle Manager/Controller Matrix Cycle/controller basic cycle 2/COMP Task - Rx_Trailer1Articulation_check/Process_Messages/Demux message CAN1 and check coherence1 ==
  CAN2_Rx_msg : Inport  OutDataTypeStr=Bus: msg_buffer_type
  expected_basic_cycle : Inport  Port=2
  Enable : EnablePort
  Bus Creator : BusCreator  Inputs=8  OutDataTypeStr=Bus: msg_buffer_type
  Bus Selector : BusSelector  OutputSignals=Buffer_1,Buffer_2,Buffer_3,Buffer_4,Buffer_5,Buffer_6,Buffer_7,Buffer_8
  Constant : Constant  Value=0  OutDataTypeStr=uint8
  Equal1 : RelationalOperator  Operator===  OutDataTypeStr=boolean  RndMeth=Simplest  InputSameDT=off
  Subsystem : Subsystem
  Terminator : Terminator
  msg_count>2_DEBUG : Subsystem
  CAN2_msg_coherent : Outport  OutputWhenDisabled=reset  InitialOutput=0  VectorParamsAs1DForOutWhenUnconnected=off
  Msg_Count_CAN2 : Outport  Port=2  VectorParamsAs1DForOutWhenUnconnected=off
  CAN2_msg : Outport  Port=3  OutDataTypeStr=Bus: msg_buffer_type  VectorParamsAs1DForOutWhenUnconnected=off
  wires:
  Bus Selector/2 -> Bus Creator/2  "<Buffer_2>"
  Bus Selector/3 -> Bus Creator/3  "<Buffer_3>"
  CAN2_Rx_msg/1 -> Bus Selector/1
  Equal1/1 -> CAN2_msg_coherent/1
  expected_basic_cycle/1 -> Equal1/2
  Bus Selector/6 -> Bus Creator/6  "<Buffer_6>"
  Bus Selector/5 -> Bus Creator/5  "<Buffer_5>"
  Bus Selector/7 -> Bus Creator/7  "<Buffer_7>"
  Bus Selector/8 -> Bus Creator/8  "<Buffer_8>"
  Bus Selector/4 -> Bus Creator/4  "<Buffer_4>"
  Bus Selector/1 -> Subsystem/1(Msg_Temporal_Data)  "<Buffer_1>"
  Subsystem/1(basic_cycle) -> Equal1/1  "basic_cycle_RX_Art1_CAN2"
  Subsystem/2(msg_count) -> Msg_Count_CAN2/1, msg_count>2_DEBUG/1(msg_c)
  Bus Creator/1 -> CAN2_msg/1
  Constant/1 -> Bus Creator/1
  Subsystem/3(board_id) -> Terminator/1

== system HANcoder_E407_TTA_Template_DS_V52/HANcoder STM32 Target - E407-STM32 algorithm/TTA CAN System/TTA System/Matrix Cycle Manager/Controller Matrix Cycle/controller basic cycle 2/COMP Task - Rx_Trailer1Articulation_check/Process_Messages/Desync calculation ==
  note: Estimation of the Local Time when the message was sent
  note: Desync CAN2
      | expected RX - Actual RX
  note: Desync CAN1
      | expected RX - Actual RX
  TM_COMM : Inport
  New_msg_CAN1 : Inport  Port=2
  msg_count_CAN1 : Inport  Port=3
  msg_count_CAN2 : Inport  Port=4
  Enable : EnablePort
  Constant : Constant  Value=COMM_Phase1
  Constant1 : Constant  Value=COMM_Phase2
  Data Store Read : DataStoreRead  DataStoreName=Msg_Rx_Ticks_CAN1  IndexOptions=Index vector (dialog)  Indices=1  OutputSizes=1
  Data Store Read1 : DataStoreRead  DataStoreName=Msg_Rx_Ticks_CAN2  IndexOptions=Index vector (dialog)  Indices=1  OutputSizes=1
  Data Store Write1 : DataStoreWrite  Priority=23  DataStoreName=Desync_Ticks  IndexOptions=Index vector (dialog)  Indices=1  OutputSizes=1
  Minus : Sum  Priority=21  Inputs=+-
  Minus1 : Sum  Priority=20  Inputs=+-
  Multiply : Product  Priority=10
  Multiply1 : Product  Priority=12
  Saturation : Saturate  UpperLimit=max_desync  LowerLimit=min_desync
  Sum : Sum  Priority=11  Inputs=+++
  Sum1 : Sum  Priority=13  Inputs=+++
  Switch1 : Switch  Priority=22  Criteria=u2 > Threshold  SaturateOnIntegerOverflow=off  InputSameDT=off
  delay_estimation_1 : Constant  Value=comm_delay_estimation1
  delay_estimation_2 : Constant  Value=comm_delay_estimation2
  wires:
  TM_COMM/1 -> Sum1/2, Sum/2
  delay_estimation_1/1 -> Sum/3
  msg_count_CAN1/1 -> Multiply/2
  Switch1/1 -> Saturation/1
  Minus/1 -> Switch1/3
  Sum1/1 -> [expected_LT_CAN2]
  delay_estimation_2/1 -> Sum1/3
  Multiply1/1 -> Sum1/1
  [expected_LT_CAN1] -> Minus1/1
  [expected_LT_CAN2] -> Minus/1
  Data Store Read1/1 -> Minus/2
  Multiply/1 -> Sum/1
  Data Store Read/1 -> Minus1/2
  msg_count_CAN2/1 -> Multiply1/2
  Sum/1 -> [expected_LT_CAN1]
  Minus1/1 -> Switch1/1
  Constant/1 -> Multiply/1
  Constant1/1 -> Multiply1/1
  New_msg_CAN1/1 -> Switch1/2
  Saturation/1 -> Data Store Write1/1  "Desync_Sync_bc2_vem_s"

== system HANcoder_E407_TTA_Template_DS_V52/HANcoder STM32 Target - E407-STM32 algorithm/TTA CAN System/TTA System/Matrix Cycle Manager/Controller Matrix Cycle/controller basic cycle 2/COMP Task - Rx_Trailer1Articulation_check/Process_Messages/Member Counter ==
  Enable : EnablePort
  AND : Logic  IconShape=distinctive  AllPortsSameDT=off  OutDataTypeStr=boolean
  AND1 : Logic  IconShape=distinctive  AllPortsSameDT=off  OutDataTypeStr=boolean
  Add : Sum
  Assign Trailer 1 as Member 1 : Subsystem
  Assign Trailer 1 as Member 2 : Subsystem
  Constant : Constant
  Constant1 : Constant
  Constant2 : Constant  Value=2
  Constant3 : Constant  Value=2
  Constant4 : Constant  Value=2
  Data Store Read : DataStoreRead  DataStoreName=Members_Nr  IndexOptions=Index vector (dialog)  Indices=1  OutputSizes=1
  Data Store Read1 : DataStoreRead  DataStoreName=Prev_Member1  IndexOptions=Index vector (dialog)  Indices=1  OutputSizes=1
  Data Store Read2 : DataStoreRead  DataStoreName=Prev_Member2  IndexOptions=Index vector (dialog)  Indices=1  OutputSizes=1
  Data Store Write : DataStoreWrite  DataStoreName=Members_Nr  IndexOptions=Index vector (dialog)  Indices=1  OutputSizes=1
  Data Store Write1 : DataStoreWrite  DataStoreName=Member_Counter_Flag  IndexOptions=Index vector (dialog)  Indices=1  OutputSizes=1
  Equal : RelationalOperator  Operator===  OutDataTypeStr=boolean  RndMeth=Simplest  InputSameDT=off
  Equal1 : RelationalOperator  Operator===  OutDataTypeStr=boolean  RndMeth=Simplest  InputSameDT=off
  NotEqual : RelationalOperator  Operator=~=  OutDataTypeStr=boolean  RndMeth=Simplest  InputSameDT=off
  NotEqual1 : RelationalOperator  Operator=~=  OutDataTypeStr=boolean  RndMeth=Simplest  InputSameDT=off
  wires:
  Data Store Read/1 -> Add/1
  Constant/1 -> Data Store Write1/1, Add/2
  Add/1 -> Equal1/1, Equal/1, Data Store Write/1
  Constant1/1 -> Equal/2
  Constant2/1 -> Equal1/2
  Data Store Read1/1 -> NotEqual/1
  Constant3/1 -> NotEqual/2
  AND/1 -> Assign Trailer 1 as Member 1/Enable
  NotEqual/1 -> AND/1
  Equal/1 -> AND/2
  AND1/1 -> Assign Trailer 1 as Member 2/Enable
  Data Store Read2/1 -> NotEqual1/1
  Constant4/1 -> NotEqual1/2
  NotEqual1/1 -> AND1/1
  Equal1/1 -> AND1/2

== system HANcoder_E407_TTA_Template_DS_V52/HANcoder STM32 Target - E407-STM32 algorithm/TTA CAN System/TTA System/Matrix Cycle Manager/Controller Matrix Cycle/controller basic cycle 2/COMP Task - Sync bc1 check/Process_Messages/Demux message CAN1 and check coherence ==
  CAN1_Rx_msg : Inport  OutDataTypeStr=Bus: msg_buffer_type
  expected_basic_cycle : Inport  Port=2
  expected_board_id : Inport  Port=3
  Enable : EnablePort
  AND : Logic  IconShape=distinctive  AllPortsSameDT=off  OutDataTypeStr=boolean
  Bus Creator : BusCreator  Inputs=8  OutDataTypeStr=Bus: msg_buffer_type
  Bus Selector : BusSelector  OutputSignals=Buffer_1,Buffer_2,Buffer_3,Buffer_4,Buffer_5,Buffer_6,Buffer_7,Buffer_8
  Constant : Constant  Value=0  OutDataTypeStr=uint8
  Equal : RelationalOperator  Operator===  OutDataTypeStr=boolean  RndMeth=Simplest  InputSameDT=off
  Equal1 : RelationalOperator  Operator===  OutDataTypeStr=boolean  RndMeth=Simplest  InputSameDT=off
  Subsystem : Subsystem
  msg_count>2_DEBUG : Subsystem
  CAN1_msg : Outport  OutDataTypeStr=Bus: msg_buffer_type  VectorParamsAs1DForOutWhenUnconnected=off
  Msg_Count_CAN1 : Outport  Port=2  VectorParamsAs1DForOutWhenUnconnected=off
  CAN1_msg_coherent : Outport  Port=3  OutputWhenDisabled=reset  InitialOutput=0  VectorParamsAs1DForOutWhenUnconnected=off
  wires:
  Bus Selector/2 -> Bus Creator/2  "<Buffer_2>"
  Bus Selector/3 -> Bus Creator/3  "<Buffer_3>"
  CAN1_Rx_msg/1 -> Bus Selector/1
  Equal/1 -> AND/2
  Equal1/1 -> AND/1
  AND/1 -> CAN1_msg_coherent/1
  expected_basic_cycle/1 -> Equal1/2
  expected_board_id/1 -> Equal/2
  Bus Selector/6 -> Bus Creator/6  "<Buffer_6>"
  Bus Selector/5 -> Bus Creator/5  "<Buffer_5>"
  Bus Selector/7 -> Bus Creator/7  "<Buffer_7>"
  Bus Selector/8 -> Bus Creator/8  "<Buffer_8>"
  Bus Selector/4 -> Bus Creator/4  "<Buffer_4>"
  Subsystem/3(board_id) -> Equal/1
  Bus Selector/1 -> Subsystem/1(Msg_Temporal_Data)  "<Buffer_1>"
  Subsystem/1(basic_cycle) -> Equal1/1
  Subsystem/2(msg_count) -> msg_count>2_DEBUG/1(msg_c), Msg_Count_CAN1/1
  Bus Creator/1 -> CAN1_msg/1
  Constant/1 -> Bus Creator/1
